simulink model "PID_CONTROLLER"  (R2021b)
settings: Solver=FixedStepDiscrete  StartTime=0.0  StopTime=50  FixedStep=0.01  RelTol=1e-3
undefined symbols (not defined in the file): kd, ki, kp, Ts, up
settings Model: Creator=sudhir  LastModifiedBy=sudhir
settings DataIOCC: SaveOutput=off  SaveTime=off
settings OptimizationCC: DefaultParameterBehavior=Inlined  GainParamInheritBuiltInType=on  UseSpecifiedMinMax=on  InlineInvariantSignals=on  EnhancedBackFolding=on  BooleansAsBitfields=on  PassReuseOutputArgsAs=Individual arguments  StateBitsets=on  DataBitsets=on  ZeroExternalMemoryAtStartup=off  ZeroInternalMemoryAtStartup=off  NoFixptDivByZeroProtection=on  LifeSpan=Auto  DifferentSizesBufferReuse=on  OptimizationPriority=RAM  OptimizationCustomize=off  EfficientTunableParamExpr=on
settings DebuggingCC: ReadBeforeWriteMsg=DisableAll  WriteAfterWriteMsg=DisableAll  WriteAfterReadMsg=DisableAll  MultiTaskDSMMsg=none  IntegerOverflowMsg=error  ParameterTunabilityLossMsg=error  IntegerSaturationMsg=error
settings ModelReferenceCC: UpdateModelReferenceTargets=IfOutOfDate
settings SFSimCC: SFSimEcho=off  MATLABDynamicMemAlloc=off
settings RTWCC: Description=Embedded Coder  SystemTargetFile=ert.tlc  GenCodeOnly=on  PackageGeneratedCodeAndArtifacts=on  PackageName=PID_CONTROLLER_CODE  TemplateMakefile=ert_default_tmf  GenerateReport=on  IncludeHyperlinkInReport=on  LaunchReport=on  GenerateTraceInfo=on  GenerateTraceReport=on  GenerateTraceReportSl=on  GenerateTraceReportSf=on  GenerateTraceReportEml=on  GenerateWebview=on  GenerateCodeMetricsReport=on  GenerateCodeReplacementReport=on
settings CodeAppCC: ForceParamTrailComments=on  IgnoreCustomStorageClasses=off  OperatorAnnotations=on  SimulinkDataObjDesc=on  SFDataObjDesc=on  InsertBlockDesc=on
settings ERTTargetCC: TargetLangStandard=C99 (ISO)  GenerateSampleERTMain=on  CombineSignalStateStructs=on  SuppressErrorStatus=on  SupportAbsoluteTime=off  SupportNonFinite=off  SupportComplex=off  ParenthesesLevel=Minimum  InlinedParameterPlacement=NonHierarchical  ERTCustomFileTemplate=example_file_process.tlc

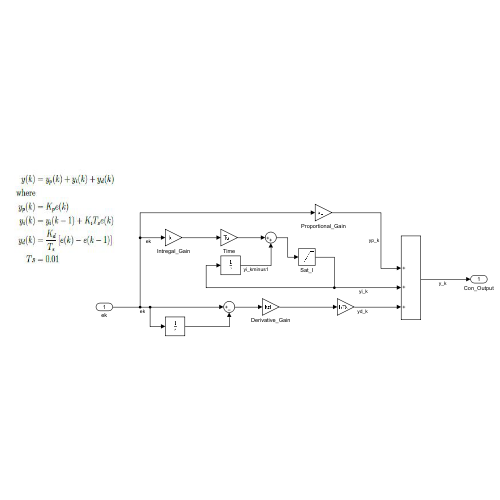
[thumbnail: Simulink's stored preview of the top-level diagram]
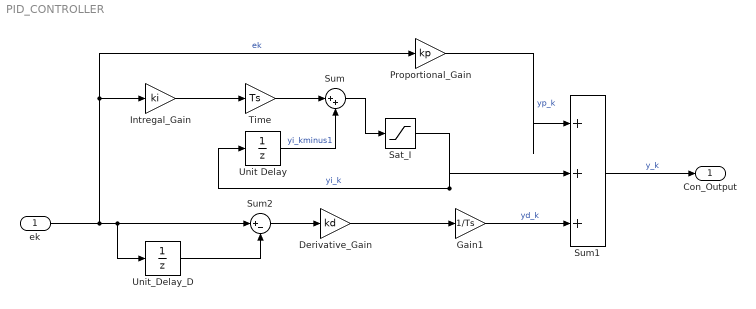
== system PID_CONTROLLER ==
  ek : Inport  OutDataTypeStr=double  PortDimensions=1  SampleTime=Ts
  Derivative_Gain : Gain  Gain=kd
  Gain1 : Gain  Gain=1/Ts
  Intregal_Gain : Gain  Gain=ki
  Proportional_Gain : Gain  Gain=kp
  Sat_I : Saturate  UpperLimit=up  LowerLimit=0
  Sum : Sum  Inputs=|++
  Sum1 : Sum  Inputs=|+++
  Sum2 : Sum  Inputs=|+-
  Time : Gain  Gain=Ts
  Unit Delay : UnitDelay  SampleTime=-1  HasFrameUpgradeWarning=on
  Unit_Delay_D : UnitDelay  SampleTime=-1  HasFrameUpgradeWarning=on
  Con_Output : Outport  OutDataTypeStr=double  PortDimensions=1  SampleTime=Ts
  wires:
  Intregal_Gain/1 -> Time/1
  Time/1 -> Sum/1
  Sum/1 -> Sat_I/1
  Gain1/1 -> Sum1/3  "yd_k"
  Proportional_Gain/1 -> Sum1/1  "yp_k"
  Unit Delay/1 -> Sum/2  "yi_kminus1"
  Sum1/1 -> Con_Output/1  "y_k"
  Derivative_Gain/1 -> Gain1/1
  Unit_Delay_D/1 -> Sum2/2
  Sum2/1 -> Derivative_Gain/1
  ek/1 -> Unit_Delay_D/1, Sum2/1, Proportional_Gain/1, Intregal_Gain/1  "ek"
  Sat_I/1 -> Unit Delay/1, Sum1/2  "yi_k"
